simulink model "prob_2"  (R2022b)
settings: Solver=VariableStepAuto  StartTime=0.0  StopTime=10.0  RelTol=1e-3
values from neighbouring files (symbols this model uses):
  b1 = 20    [problem_2.m]
  b2 = 20    [problem_2.m]
  k1 = 50    [problem_2.m]
  k2 = 5    [problem_2.m]
  m1 = 2    [problem_2.m]
  m2 = 10    [problem_2.m]
settings Model: Creator=adnzw  LastModifiedBy=adnzw

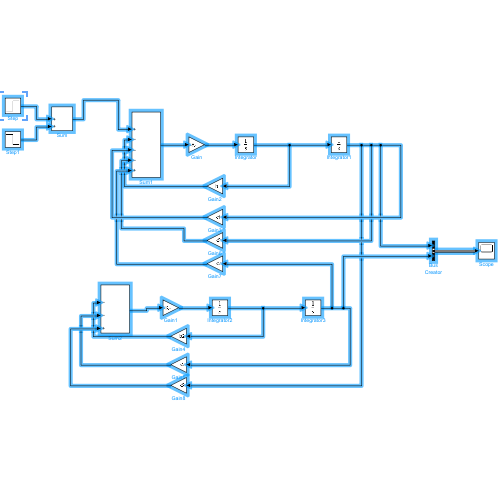
[thumbnail: Simulink's stored preview of the top-level diagram]
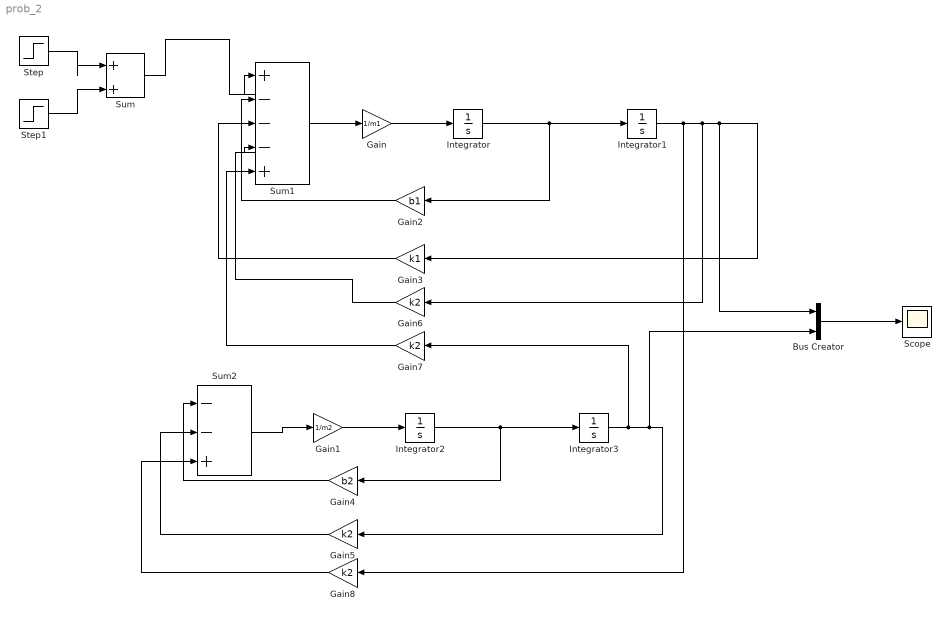
== system prob_2 ==
  Bus Creator : BusCreator  Inputs=2
  Gain : Gain  Gain=1/m1
  Gain1 : Gain  Gain=1/m2
  Gain2 : Gain  Gain=b1
  Gain3 : Gain  Gain=k1
  Gain4 : Gain  Gain=b2
  Gain{5..8} (4 alike) : Gain  Gain=k2
  Integrator{,1..3} (4 alike) : Integrator
  Scope : Scope
  Step : Step  After=100  SampleTime=0
  Step1 : Step  Time=5  After=-100  SampleTime=0
  Sum : Sum  Inputs=|++
  Sum1 : Sum  Inputs=|+---+
  Sum2 : Sum  Inputs=|--+
  wires:
  Step/1 -> Sum/1
  Step1/1 -> Sum/2
  Sum/1 -> Sum1/1
  Sum1/1 -> Gain/1
  Integrator/1 -> Gain2/1, Integrator1/1
  Sum2/1 -> Gain1/1
  Integrator2/1 -> Gain4/1, Integrator3/1
  Gain/1 -> Integrator/1
  Gain1/1 -> Integrator2/1
  Integrator1/1 -> Gain8/1, Gain6/1, Bus Creator/1, Gain3/1
  Integrator3/1 -> Gain7/1, Bus Creator/2, Gain5/1
  Gain2/1 -> Sum1/2
  Gain3/1 -> Sum1/3
  Gain6/1 -> Sum1/4
  Gain4/1 -> Sum2/1
  Gain5/1 -> Sum2/2
  Gain7/1 -> Sum1/5
  Gain8/1 -> Sum2/3
  Bus Creator/1 -> Scope/1
